simulink model "gpio_ctrl"  (Simulink 6.2)
settings: Solver=ode45  StartTime=0.0  StopTime=100  RelTol=1e-3
libraries: xps_library x4, xbsIndex_r3 x2
settings Model: LastModifiedBy=wjm
settings DebuggingCC: SolverPrmCheckMsg=warning

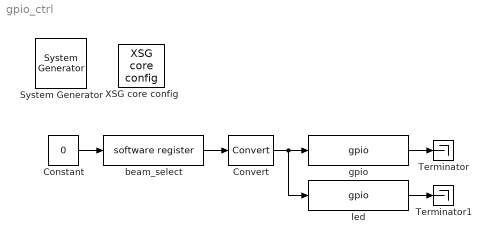
== system gpio_ctrl ==
  " System Generator" : xbsIndex_r3/ System Generator  Tag=genX  xilinxfamily=Virtex2P  part=xc2vp50  speed=-7  package=ff1152  synthesis_tool=XST  directory=./gpio_ctrl/sysgen  testbench=off  simulink_period=1  sysclk_period=10  incr_netlist=off  trim_vbits=Everywhere in SubSystem  dbl_ovrd=According to Block Masks  core_generation=According to Block Masks  run_coregen=off  deprecated_control=off  eval_field=0
      settings: AttributesFormatString=System\nGenerator
  Constant : Constant  Value=0  VectorParams1D=off  SampleTime=1
  Convert : xbsIndex_r3/Convert  arith_type=Unsigned  n_bits=8  bin_pt=0  quantization=Truncate  overflow=Wrap  latency=1  explicit_period=on  period=1  dbl_ovrd=off  show_param=off  inserted_by_tool=off  pipeline=off
      settings: xl_area=[0, 0, 0, 0, 0, 0, 0]
  Terminator : Terminator
  Terminator1 : Terminator
  XSG core config : xps_library/XSG core config  Tag=xps:xsg  hw_sys=iBOB  ibob_linux=off  clk_src=sys_clk  gpio_clk_io_group=iBOB:sma  gpio_clk_bit_index=0  clk_rate=100  sample_period=1  synthesis_tool=XST  mpc_type=powerpc405
  beam_select : xps_library/software register  Tag=xps:sw_reg  io_dir=From Processor  arith_type=Unsigned  bitwidth=32  bin_pt=0  sample_period=1  gw_name=gpio_ctrl_beam_select_user_data_out
  gpio : xps_library/gpio  Tag=xps:gpio  io_group=iBOB:gpio0  io_dir=out  arith_type=Unsigned  bitwidth=8  bin_pt=0  bit_index=[0:7]  sample_period=1  use_single_ended=off  use_ddr=off  reg_iob=off  reg_clk_phase=0  termination=None
  led : xps_library/gpio  Tag=xps:gpio  io_group=iBOB:led  io_dir=out  arith_type=Unsigned  bitwidth=8  bin_pt=0  bit_index=[0:7]  sample_period=1  use_single_ended=off  use_ddr=off  reg_iob=off  reg_clk_phase=0  termination=None
  wires:
  Constant/1 -> beam_select/1
  beam_select/1 -> Convert/1
  gpio/1 -> Terminator/1
  led/1 -> Terminator1/1
  Convert/1 -> gpio/1, led/1
